simulink model "model2_tm"  (R2018b)
settings: Solver=ode8  StartTime=0.0  StopTime=Inf  FixedStep=0.01  RelTol=1e-3  EnableMultiTasking=on
StopFcn:
  | stopCallback
values from neighbouring files (symbols this model uses):
  params = 1.0    [testModel2_td.sldd]
undefined symbols (not defined in the file or in its folder): ipaddr, PTP
libraries: slrtlib x5, filteredPDController_ul x3, xpcutilitieslib x3, ptplib x3, xpcrtudplib x3, find6DOF_cl x1, outputCommands_ul x1, risingDebounce_ul x1, manualMotorOverride x1
settings Model: DataDictionary=testModel2_td.sldd  sg_rtwmakecfg_data=_sglibc_  Creator=mcobb  LastModifiedBy=Cole
settings SolverCC: ConcurrentTasks=on  AutoInsertRateTranBlk=on
settings DataIOCC: SaveFormat=StructureWithTime
settings OptimizationCC: BlockReduction=off  OptimizeBlockIOStorage=off  BufferReuse=off  GlobalBufferReuse=off  ExpressionFolding=off  LocalBlockOutputs=off  OptimizeDataStoreBuffers=off  BusAssignmentInplaceUpdate=off
settings DebuggingCC: ParameterOverflowMsg=none  LibraryContextMissingDiagnostic=none
settings HardwareCC: ProdBitPerPointer=32  ProdBitPerSizeT=32  ProdBitPerPtrDiffT=32  ProdLargestAtomicFloat=None  ProdWordSize=32  ProdLongLongMode=on  ProdHWDeviceType=Generic->32-bit x86 compatible
settings SFSimCC: SimUseLocalCustomCode=off
settings RTWCC: SystemTargetFile=slrt.tlc  TemplateMakefile=slrt_default_tmf  Description=Simulink Real-Time  RTWUseLocalCustomCode=off  CodeExecutionProfiling=on  RTWCompilerOptimization=on
settings SimulinkRealTimeCC: SupportVariableSizeSignals=on  PreserveStateflowLocalDataDimensions=off  RL32LogTETModifier=off  xPCConcurrentTasks=on

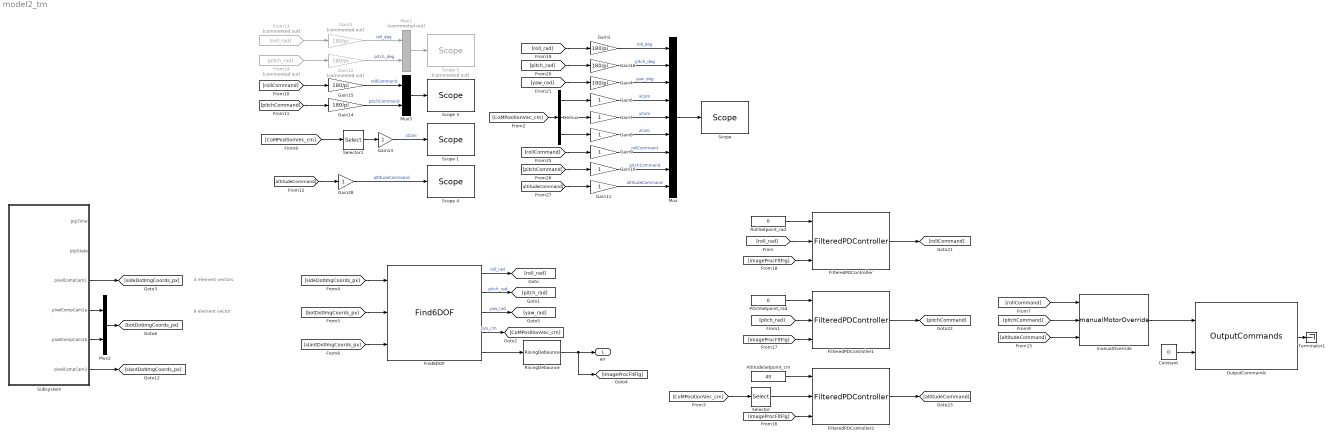
== system model2_tm ==
  note: 8 element vector
  note: 4 element vectors
  AltitudeSetpoint_cm : Constant  Value=40
  Constant : Constant  Value=0
  Demux : Demux  Outputs=3
  FilteredPDController : filteredPDController_ul/FilteredPDController  enable=on  kp=params.rollCtrlkp_Prad.Value  kd=params.rollCtrlkd_sPrad.Value  timeConstant_s=params.rollCtrltau_s.Value  intialError=0  initialOutput=0
  FilteredPDController1 : filteredPDController_ul/FilteredPDController  enable=on  kp=params.pitchCtrlkp_Prad.Value  kd=params.pitchCtrlkd_sPrad.Value  timeConstant_s=params.pitchCtrltau_s.Value  intialError=0  initialOutput=0
  FilteredPDController2 : filteredPDController_ul/FilteredPDController  enable=on  kp=params.altCtrlkp_Prad.Value  kd=params.altCtrlkd_sPrad.Value  timeConstant_s=params.altCtrltau_s.Value  intialError=0  initialOutput=0
  Find6DOF : find6DOF_cl/Find6DOF  imageDims_px=params.sideImageSize_px.Value  initialCoMPositionVec_cm=params.initCoMPosVec_cm.Value  cameraFOVAngles_deg=params.cameraFOV_deg.Value  sideEulerAngles=params.sideCamEulAng_deg.Value  sideCamPositionVec_cm=params.sideCamPosVec_cm.Value  botEulerAngles=params.botCamEulAng_deg.Value  botCamPositionVec_cm=params.botCamPosVec_cm.Value  slantEulerAngles=params.slntCamEulAng_deg.Value  slantCamPositionVec_cm=params.slntCamPosVec_cm.Value  sideSeparation_cm=params.sideDotSepDist_cm.Value  sidePositionVecBF_cm=params.sideDotPosVec_cm.Value  bottomASeparation_cm=params.botADotSepDist_cm.Value  botAPositionVecBF_cm=params.botADotPosVec_cm.Value  bottomBSeparation_cm=params.botBDotSepDist_cm.Value  botBPositionVecBG_cm=params.botBDotPosVec_cm.Value
  From13 : From  Commented=on  GotoTag=roll_rad
  From14 : From  Commented=on  GotoTag=pitch_rad
  Gain{6..11,13,28} (8 alike) : Gain
  Gain12 : Gain  Commented=on  Gain=180/pi
  Gain{3..4,14..16} (5 alike) : Gain  Gain=180/pi
  Gain5 : Gain  Commented=on  Gain=180/pi
  Mux : Mux  Inputs=9
  Mux1 : Mux  Commented=on  Inputs=2
  Mux2 : Mux  Inputs=2
  Mux5 : Mux  Inputs=2
  OutputCommands : outputCommands_ul/OutputCommands  maxVoltage=params.maxOutVltg_vlt.Value
  PitchSetpoint_rad : Constant  Value=0
  RisingDebounce : risingDebounce_ul/RisingDebounce  threshold=params.imagProcErrThrsh_na.Value  timeDelay_s=params.imagProcErrDbncTm_s.Value
  RollSetpoint_rad : Constant  Value=0
  "Scope " : slrtlib/Displays and Logging/Scope   scopeno=1  scopetype=Target  autostart=on  viewmode=Numerical  formatstr='%15.6f'  grid=on  ylimits=[0,0]  nosamples=250  noprepostsamples=0  interleave=1  triggermode=FreeRun  triggersignal=1  trigsignalfromport=off  triggerlevel=0.0  triggerslope=Either  triggerscope=1  triggersample=0  filename=data.dat  mode=Lazy  writesize=512  autorestart=off  dynamicfilemode=off  maxwritefilesize=512*1024^2
  Scope 1 : slrtlib/Displays and Logging/Scope   scopeno=3  scopetype=Target  autostart=on  viewmode=Graphical rolling  formatstr='%15.6f'  grid=on  ylimits=[0,50]  nosamples=1000  noprepostsamples=0  interleave=1  triggermode=FreeRun  triggersignal=1  trigsignalfromport=off  triggerlevel=0.0  triggerslope=Either  triggerscope=1  triggersample=0  filename=data.dat  mode=Lazy  writesize=512  autorestart=off  dynamicfilemode=off  maxwritefilesize=512*1024^2
  Scope 3 : slrtlib/Displays and Logging/Scope   scopeno=2  scopetype=Target  autostart=on  viewmode=Graphical rolling  formatstr='%15.6f'  grid=on  ylimits=[-30,30]  nosamples=1000  noprepostsamples=0  interleave=1  triggermode=FreeRun  triggersignal=1  trigsignalfromport=off  triggerlevel=0.0  triggerslope=Either  triggerscope=1  triggersample=0  filename=data.dat  mode=Lazy  writesize=512  autorestart=off  dynamicfilemode=off  maxwritefilesize=512*1024^2
  Scope 4 : slrtlib/Displays and Logging/Scope   scopeno=4  scopetype=Target  autostart=on  viewmode=Graphical rolling  formatstr='%15.6f'  grid=on  ylimits=[-50,0]  nosamples=1000  noprepostsamples=0  interleave=1  triggermode=FreeRun  triggersignal=1  trigsignalfromport=off  triggerlevel=0.0  triggerslope=Either  triggerscope=1  triggersample=0  filename=data.dat  mode=Lazy  writesize=512  autorestart=off  dynamicfilemode=off  maxwritefilesize=512*1024^2
  Scope 5 : slrtlib/Displays and Logging/Scope   Commented=on  scopeno=1  scopetype=Target  autostart=on  viewmode=Graphical rolling  formatstr='%15.6f'  grid=on  ylimits=[-30,30]  nosamples=1000  noprepostsamples=0  interleave=1  triggermode=FreeRun  triggersignal=1  trigsignalfromport=off  triggerlevel=0.0  triggerslope=Either  triggerscope=1  triggersample=0  filename=data.dat  mode=Lazy  writesize=512  autorestart=off  dynamicfilemode=off  maxwritefilesize=512*1024^2
  Selector : Selector  InputPortWidth=3  IndexOptions=Index vector (dialog)  Indices=3  OutputSizes=1
  Selector1 : Selector  InputPortWidth=3  IndexOptions=Index vector (dialog)  Indices=3  OutputSizes=1
  Subsystem : Subsystem  TreatAsAtomicUnit=on  mask{sample_time=0.01, announce_interval=params.announceInterval_s.Value, sync_interval=params.syncInterval_s.Value}
      mask prompts: sample_time "Sample time (-1 for inherited)"; announce_interval "Announce interval (second):"; sync_interval "Sync interval (second):"
      mask TypeOptions sample_time: IEEE 1588 Read State/sample_time | IEEE 1588 Read Time/sample_time | IEEE 1588 Real-Time UDP/sample_time | UDP Receive Machine 3/sampleTime | UDP Receive Machine 4/sampleTime | UDP Receive Machine 5/sampleTime
      mask TypeOptions announce_interval: IEEE 1588 Real-Time UDP/announce_interval
      mask TypeOptions sync_interval: IEEE 1588 Real-Time UDP/sync_interval
  Terminator1 : Terminator
  manualOverride : manualMotorOverride/manualMotorOverride  enbl=off  mtr1CmdOvrrd=params.mtr1ManulaSpdCmd_na.Value  mtr2CmdOvrrd=params.mtr2ManulaSpdCmd_na.Value  mtr3CmdOvrrd=params.mtr3ManulaSpdCmd_na.Value
  err : Outport
  wires:
  FilteredPDController/1 -> [rollCommand]
  [roll_rad] -> FilteredPDController/2
  RollSetpoint_rad/1 -> FilteredPDController/1
  FilteredPDController1/1 -> [pitchCommand]
  FilteredPDController2/1 -> [altitudeCommand]
  PitchSetpoint_rad/1 -> FilteredPDController1/1
  [pitch_rad] -> FilteredPDController1/2
  AltitudeSetpoint_cm/1 -> FilteredPDController2/1
  Subsystem/3(pixelCompCam1) -> [sideDotImgCoords_px]
  Subsystem/6(pixelCompCam3) -> [slantDotImgCoords_px]
  Selector/1 -> FilteredPDController2/2
  [yaw_rad] -> Gain4/1
  [pitch_rad] -> Gain16/1
  [roll_rad] -> Gain3/1
  Demux/1 -> Gain6/1
  Demux/2 -> Gain7/1
  Gain4/1 -> Mux/3  "yaw_deg"
  Gain16/1 -> Mux/2  "pitch_deg"
  Gain3/1 -> Mux/1  "roll_deg"
  Demux/3 -> Gain8/1
  [rollCommand] -> Gain9/1
  [pitchCommand] -> Gain10/1
  [altitudeCommand] -> Gain11/1
  Mux/1 -> "Scope "/1
  Gain6/1 -> Mux/4  "xCom"
  Gain7/1 -> Mux/5  "yCom"
  Gain8/1 -> Mux/6  "zCom"
  Gain9/1 -> Mux/7  "rollCommand"
  Gain10/1 -> Mux/8  "pitchCommand"
  Gain11/1 -> Mux/9  "altitudeCommand"
  Mux5/1 -> Scope 3/1
  Gain28/1 -> Scope 4/1  "altitudeCommand"
  [altitudeCommand] -> Gain28/1
  Find6DOF/1 -> [roll_rad]  "roll_rad"
  Find6DOF/2 -> [pitch_rad]  "pitch_rad"
  Find6DOF/3 -> [yaw_rad]  "yaw_rad"
  Find6DOF/4 -> [CoMPositionVec_cm]  "pos_cm"
  [CoMPositionVec_cm] -> Demux/1
  [CoMPositionVec_cm] -> Selector/1
  Constant/1 -> OutputCommands/2
  [sideDotImgCoords_px] -> Find6DOF/1
  [botDotImgCoords_px] -> Find6DOF/2
  [slantDotImgCoords_px] -> Find6DOF/3
  Mux2/1 -> [botDotImgCoords_px]
  Subsystem/5(pixelCompCam2b) -> Mux2/2
  Subsystem/4(pixelCompCam2a) -> Mux2/1
  Gain12/1 -> Mux1/2  "pitch_deg"
  Gain5/1 -> Mux1/1  "roll_deg"
  Mux1/1 -> Scope 5/1
  From13/1 -> Gain5/1
  From14/1 -> Gain12/1
  [CoMPositionVec_cm] -> Selector1/1
  Selector1/1 -> Gain13/1
  Gain13/1 -> Scope 1/1  "zCom"
  [pitchCommand] -> Gain14/1
  [rollCommand] -> Gain15/1
  Gain15/1 -> Mux5/1  "rollCommand"
  Gain14/1 -> Mux5/2  "pitchCommand"
  Find6DOF/5 -> RisingDebounce/1
  RisingDebounce/1 -> [imageProcFltFlg], err/1
  [rollCommand] -> manualOverride/1
  [pitchCommand] -> manualOverride/2
  [altitudeCommand] -> manualOverride/3
  manualOverride/1 -> OutputCommands/1
  [imageProcFltFlg] -> FilteredPDController2/3
  [imageProcFltFlg] -> FilteredPDController1/3
  [imageProcFltFlg] -> FilteredPDController/3
  OutputCommands/1 -> Terminator1/1

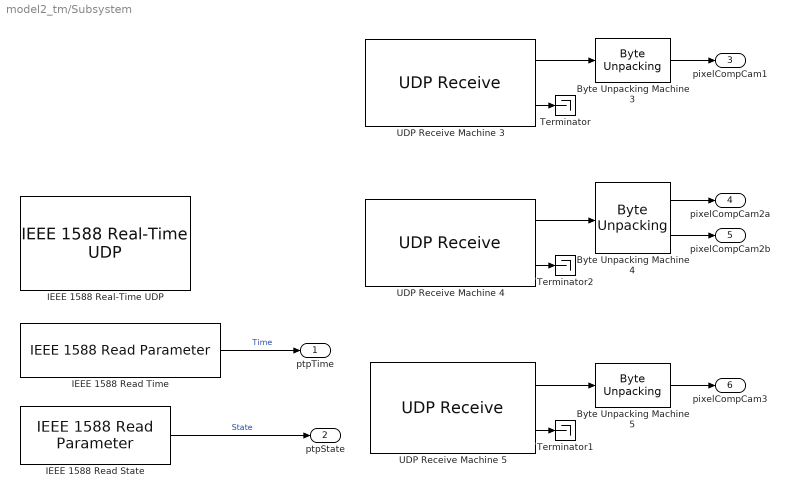
== system model2_tm/Subsystem ==
  "Byte Unpacking Machine 3 " : xpcutilitieslib/Byte Unpacking   MaskUnpackedDataTypes={['double']}  MaskUnpackedDataSizes={[4]}  MaskAlignment=1
      settings: SourceProductName=Simulink Real-Time  SourceProductBaseCode=XP
  Byte Unpacking Machine 4 : xpcutilitieslib/Byte Unpacking   MaskUnpackedDataTypes={['double'],['double']}  MaskUnpackedDataSizes={[4],[4]}  MaskAlignment=1
      settings: SourceProductName=Simulink Real-Time  SourceProductBaseCode=XP
  Byte Unpacking Machine 5 : xpcutilitieslib/Byte Unpacking   MaskUnpackedDataTypes={['double']}  MaskUnpackedDataSizes={[4]}  MaskAlignment=1
      settings: SourceProductName=Simulink Real-Time  SourceProductBaseCode=XP
  IEEE 1588 Read State : ptplib/IEEE 1588 Read Parameter  Priority=1  ID=1  param=Protocol state  sample_time=sample_time  enable_read_precision=off
      settings: SourceProductName=Simulink Real-Time  SourceProductBaseCode=XP
  IEEE 1588 Read Time : ptplib/IEEE 1588 Read Parameter  Priority=1  ID=1  param=PTP time (time-of-day)  sample_time=sample_time  enable_read_precision=off
      settings: SourceProductName=Simulink Real-Time  SourceProductBaseCode=XP
  IEEE 1588 Real-Time UDP : ptplib/IEEE 1588 Real-Time UDP  Priority=0  ID=1  PciBus=2  PciSlot=0  PciFunction=0  time_inc=4000000  sample_time=sample_time  IpSource=Specify  IpAddress=30.30.30.30  SubnetMask=255.255.255.0  Gateway=0.0.0.0  Receive1=0.0.0.0  dest_ip_select=Specify  custom_dest_ip_addr=255.255.255.255  MulticastList=[ipaddr('224.0.1.129'), ipaddr('224.0.0.107')]  Multicast={macaddr('01:00:5E:00:01:81'), macaddr('01:00:5E:00:00:6B')}  time_source=Ethernet board  timescale=PTP (1970-01-01)  epoch=[1970 01 01 00]  delay_measure=Request-response  slave_only=off  enable_advanced_config=on  domain_num=0  utc_offset=35  priority1=1  clock_class=248  clock_accuracy=hex2dec('FE')  priority2=1  announce_interval=announce_interval  sync_interval=sync_interval  min_pdelay_req_interval=2  announce_receipt_timeout=30
      settings: SourceProductName=Simulink Real-Time  SourceProductBaseCode=XP
  Terminator : Terminator
  Terminator1 : Terminator
  Terminator2 : Terminator
  UDP Receive Machine 3 : xpcrtudplib/UDP Receive  ipAddressVal=30.30.30.30  localPort=8001  rcvWidth=32  rcvFmAny=off  fmAddress=30.30.30.1  rcvMulticast=off  multicastAddress={30.30.30.1, 30.30.30.2, 30.30.30.3}  maxUDPQueue=8  sampleTime=sample_time
      settings: SourceProductName=Simulink Real-Time
  UDP Receive Machine 4 : xpcrtudplib/UDP Receive  ipAddressVal=30.30.30.30  localPort=8002  rcvWidth=64  rcvFmAny=off  fmAddress=30.30.30.2  rcvMulticast=off  multicastAddress={30.30.30.1, 30.30.30.2, 30.30.30.3}  maxUDPQueue=8  sampleTime=sample_time
      settings: SourceProductName=Simulink Real-Time
  UDP Receive Machine 5 : xpcrtudplib/UDP Receive  ipAddressVal=30.30.30.30  localPort=8003  rcvWidth=32  rcvFmAny=off  fmAddress=30.30.30.3  rcvMulticast=off  multicastAddress={30.30.30.1, 30.30.30.2, 30.30.30.3}  maxUDPQueue=8  sampleTime=sample_time
      settings: SourceProductName=Simulink Real-Time
  ptpTime : Outport
  ptpState : Outport  Port=2
  pixelCompCam1 : Outport  Port=3
  pixelCompCam2a : Outport  Port=4
  pixelCompCam2b : Outport  Port=5
  pixelCompCam3 : Outport  Port=6
  wires:
  UDP Receive Machine 3/1 -> "Byte Unpacking Machine 3 "/1
  UDP Receive Machine 4/1 -> Byte Unpacking Machine 4/1
  IEEE 1588 Read Time/1 -> ptpTime/1  "Time"
  UDP Receive Machine 3/2 -> Terminator/1
  UDP Receive Machine 5/2 -> Terminator1/1
  "Byte Unpacking Machine 3 "/1 -> pixelCompCam1/1
  UDP Receive Machine 4/2 -> Terminator2/1
  Byte Unpacking Machine 5/1 -> pixelCompCam3/1
  IEEE 1588 Read State/1 -> ptpState/1  "State"
  UDP Receive Machine 5/1 -> Byte Unpacking Machine 5/1
  Byte Unpacking Machine 4/1 -> pixelCompCam2a/1
  Byte Unpacking Machine 4/2 -> pixelCompCam2b/1
